simulink model "Task7"  (R2022a)
settings: Solver=FixedStepAuto  StartTime=0.0  StopTime=23  FixedStep=0.001  RelTol=1e-3
undefined symbols (not defined in the file): q, WrDenSol, WrNumSol
settings Model: Creator=Family  LastModifiedBy=Family

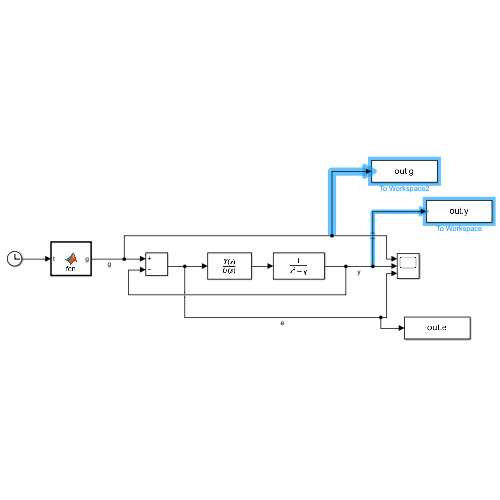
[thumbnail: Simulink's stored preview of the top-level diagram]
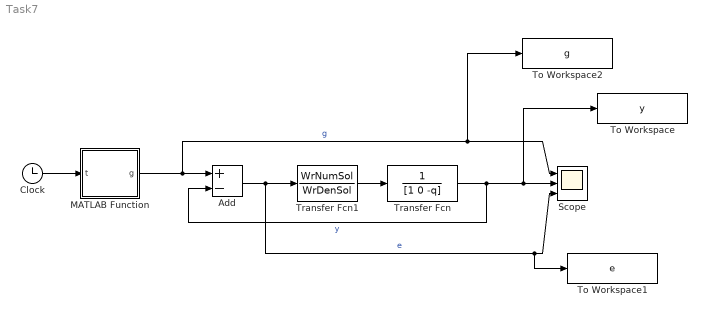
== system Task7 ==
  Add : Sum  Inputs=+-
  Clock : Clock
  MATLAB Function : MATLAB Function  TreatAsAtomicUnit=on
  Scope : Scope  NumInputPorts=3
  To Workspace : ToWorkspace  VariableName=y  SaveFormat=Timeseries  SampleTime=-1
  To Workspace1 : ToWorkspace  VariableName=e  SaveFormat=Timeseries  SampleTime=-1
  To Workspace2 : ToWorkspace  VariableName=g  SaveFormat=Timeseries  SampleTime=-1
  Transfer Fcn : TransferFcn  Denominator=[1 0 -q]
  Transfer Fcn1 : TransferFcn  Numerator=WrNumSol  Denominator=WrDenSol
  wires:
  Transfer Fcn/1 -> Add/2, To Workspace/1, Scope/2  "y"
  Add/1 -> Transfer Fcn1/1, To Workspace1/1, Scope/3  "e"
  Transfer Fcn1/1 -> Transfer Fcn/1
  Clock/1 -> MATLAB Function/1(t)
  MATLAB Function/1(g) -> To Workspace2/1, Scope/1, Add/1  "g"

== matlab function Task7/MATLAB Function ==
  data: t input; g output
function g = fcn(t)

g = 2*sin(3*t);
